simulink model "PRACTICA4"  (R2015a)
settings: Solver=ode4  StartTime=0.0  StopTime=10  FixedStep=1e-3  RelTol=1e-3
libraries: simulink x2
settings Model: Creator=exeld  LastModifiedBy=exeld

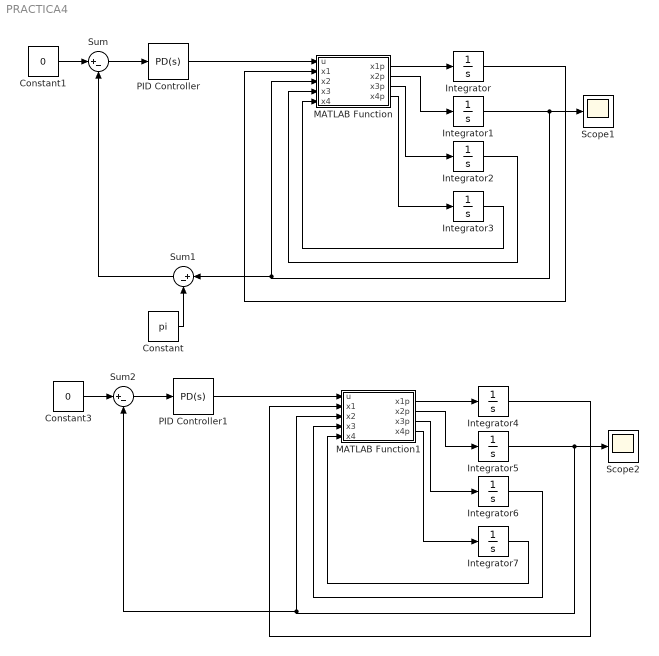
== system PRACTICA4 ==
  Constant : Constant  Value=pi
  Constant1 : Constant  Value=0
  Constant3 : Constant  Value=0
  Integrator{,2..4,6..7} (6 alike) : Integrator
  Integrator1 : Integrator  InitialCondition=pi+0.4
  Integrator5 : Integrator  InitialCondition=0.1
  MATLAB Function : MATLAB Function  TreatAsAtomicUnit=on
  MATLAB Function1 : MATLAB Function  TreatAsAtomicUnit=on
  PID Controller : simulink/Continuous/PID Controller  Controller=PD  TimeDomain=Continuous-time  SampleTime=-1  IntegratorMethod=Forward Euler  FilterMethod=Forward Euler  Form=Parallel  UseFilter=on  ControllerParametersSource=internal  P=4.007  I=0  D=0.959  N=100  InitialConditionSource=internal  InitialConditionForIntegrator=0  InitialConditionForFilter=0  ExternalReset=none  LimitOutput=off  UpperSaturationLimit=inf  LowerSaturationLimit=-inf  LinearizeAsGain=on  AntiWindupMode=none  Kb=1  TrackingMode=off  Kt=1  PParamMin=[]  PParamMax=[]  IParamMin=[]  IParamMax=[]  DParamMin=[]  DParamMax=[]  NParamMin=[]  NParamMax=[]  KbParamMin=[]  KbParamMax=[]  KtParamMin=[]  KtParamMax=[]  POutMin=[]  POutMax=[]  IOutMin=[]  IOutMax=[]  DOutMin=[]  DOutMax=[]  NOutMin=[]  NOutMax=[]  KbOutMin=[]  KbOutMax=[]  KtOutMin=[]  KtOutMax=[]  IntegratorOutMin=[]  IntegratorOutMax=[]  FilterOutMin=[]  FilterOutMax=[]  SumOutMin=[]  SumOutMax=[]  SumI1OutMin=[]  SumI1OutMax=[]  SumI2OutMin=[]  SumI2OutMax=[]  SumI3OutMin=[]  SumI3OutMax=[]  SumDOutMin=[]  SumDOutMax=[]  SaturationOutMin=[]  SaturationOutMax=[]  IntegratorContinuousStateAttributes=''  IntegratorStateMustResolveToSignalObject=off  IntegratorRTWStateStorageClass=Auto  FilterContinuousStateAttributes=''  FilterStateMustResolveToSignalObject=off  FilterRTWStateStorageClass=Auto  DifferentiatorICPrevScaledInput=0  DifferentiatorOutMin=[]  DifferentiatorOutMax=[]
  PID Controller1 : simulink/Continuous/PID Controller  Controller=PD  TimeDomain=Continuous-time  SampleTime=-1  IntegratorMethod=Forward Euler  FilterMethod=Forward Euler  Form=Parallel  UseFilter=on  ControllerParametersSource=internal  P=-24.612  I=0  D=-1.6  N=100  InitialConditionSource=internal  InitialConditionForIntegrator=0  InitialConditionForFilter=0  ExternalReset=none  LimitOutput=off  UpperSaturationLimit=inf  LowerSaturationLimit=-inf  LinearizeAsGain=on  AntiWindupMode=none  Kb=1  TrackingMode=off  Kt=1  PParamMin=[]  PParamMax=[]  IParamMin=[]  IParamMax=[]  DParamMin=[]  DParamMax=[]  NParamMin=[]  NParamMax=[]  KbParamMin=[]  KbParamMax=[]  KtParamMin=[]  KtParamMax=[]  POutMin=[]  POutMax=[]  IOutMin=[]  IOutMax=[]  DOutMin=[]  DOutMax=[]  NOutMin=[]  NOutMax=[]  KbOutMin=[]  KbOutMax=[]  KtOutMin=[]  KtOutMax=[]  IntegratorOutMin=[]  IntegratorOutMax=[]  FilterOutMin=[]  FilterOutMax=[]  SumOutMin=[]  SumOutMax=[]  SumI1OutMin=[]  SumI1OutMax=[]  SumI2OutMin=[]  SumI2OutMax=[]  SumI3OutMin=[]  SumI3OutMax=[]  SumDOutMin=[]  SumDOutMax=[]  SaturationOutMin=[]  SaturationOutMax=[]  IntegratorContinuousStateAttributes=''  IntegratorStateMustResolveToSignalObject=off  IntegratorRTWStateStorageClass=Auto  FilterContinuousStateAttributes=''  FilterStateMustResolveToSignalObject=off  FilterRTWStateStorageClass=Auto  DifferentiatorICPrevScaledInput=0  DifferentiatorOutMin=[]  DifferentiatorOutMax=[]
  Scope1 : Scope
      settings: YMin=3.04  YMax=3.22
  Scope2 : Scope
      settings: YMin=3.04  YMax=3.22
  Sum : Sum  Inputs=|+-
  Sum1 : Sum  Inputs=|+-
  Sum2 : Sum  Inputs=|+-
  wires:
  MATLAB Function/1(x1p) -> Integrator/1
  MATLAB Function/2(x2p) -> Integrator1/1
  MATLAB Function/3(x3p) -> Integrator2/1
  MATLAB Function/4(x4p) -> Integrator3/1
  Integrator/1 -> MATLAB Function/2(x1)
  Integrator3/1 -> MATLAB Function/5(x4)
  Integrator2/1 -> MATLAB Function/4(x3)
  Integrator1/1 -> Scope1/1, MATLAB Function/3(x2), Sum1/1
  Constant/1 -> Sum1/2
  Sum1/1 -> Sum/2
  Constant1/1 -> Sum/1
  Sum/1 -> PID Controller/1
  PID Controller/1 -> MATLAB Function/1(u)
  MATLAB Function1/1(x1p) -> Integrator4/1
  MATLAB Function1/2(x2p) -> Integrator5/1
  MATLAB Function1/3(x3p) -> Integrator6/1
  MATLAB Function1/4(x4p) -> Integrator7/1
  Integrator4/1 -> MATLAB Function1/2(x1)
  Integrator7/1 -> MATLAB Function1/5(x4)
  Integrator6/1 -> MATLAB Function1/4(x3)
  Integrator5/1 -> Scope2/1, Sum2/2, MATLAB Function1/3(x2)
  Constant3/1 -> Sum2/1
  Sum2/1 -> PID Controller1/1
  PID Controller1/1 -> MATLAB Function1/1(u)

== matlab function PRACTICA4/MATLAB Function1 ==
  data: u input; x1p output; x1 input; x2 input; x3 input; x4 input; x2p output; x3p output; x4p output
function [x1p,x2p,x3p,x4p] = fcn(u,x1,x2,x3,x4)
l=.3;
m=.1;
M=.2;
b1=.01;
b2=.01;
g=9.81;
fx=[x3;x4;1/(l*(M+m-(m*cos(x2)^2)))*((b2*x4*cos(x2))+(l^2*m*x4^2*sin(x2))-(l*b1*x3)-(l*m*g*cos(x2)*sin(x2)));1/(l^2*m*(M+m-(m*cos(x2)^2)))*(-((M+m)*(b2*x4-l*g*m*sin(x2)))-(l*m*cos(x2)*(l*m*x4^2*sin(x2)-b1*x3)))];
gx=[0;0;1/(M+m*(sin(x2)^2));-(cos(x2))/(l*(M+m*(sin(x2)^2)))];
xx=fx+gx*u;
x1p=xx(1,1);
x2p=xx(2,1);
x3p=xx(3,1);
x4p=xx(4,1);

== matlab function PRACTICA4/MATLAB Function ==
  data: u input; x1p output; x1 input; x2 input; x3 input; x4 input; x2p output; x3p output; x4p output
function [x1p,x2p,x3p,x4p] = fcn(u,x1,x2,x3,x4)
l=.3;
m=.1;
M=.2;
b1=.01;
b2=.01;
g=9.81;
fx=[x3;x4;1/(l*(M+m-(m*cos(x2)^2)))*((b2*x4*cos(x2))+(l^2*m*x4^2*sin(x2))-(l*b1*x3)-(l*m*g*cos(x2)*sin(x2)));1/(l^2*m*(M+m-(m*cos(x2)^2)))*(-((M+m)*(b2*x4-l*g*m*sin(x2)))-(l*m*cos(x2)*(l*m*x4^2*sin(x2)-b1*x3)))];
gx=[0;0;1/(M+m*(sin(x2)^2));-(cos(x2))/(l*(M+m*(sin(x2)^2)))];
xx=fx+gx*u;
x1p=xx(1,1);
x2p=xx(2,1);
x3p=xx(3,1);
x4p=xx(4,1);
